simulink model "Tractor_KRAKER_etrailer_v1_2023a"  (R2023a)
settings: Solver=VariableStepAuto  StartTime=0.0  StopTime=tmax  FixedStep=dt  RelTol=1e-3  EnableMultiTasking=on
PreLoadFcn:
  | init_vehicle
  | SIMSCAPE_BE_driveline_etrailer_parameters
StartFcn:
  | tic
StopFcn:
  | toc
  | sim_stop_function
  | Etrailer_Simscape_MBM_plotting
undefined symbols (not defined in the file): brake_input, chassis_length, end_val, energyCapacity, final_x, final_y, Floor, front_overhang, initialSOC, InputSwitch, kI, L_0f, LD, mass_trailer, massload, MaxTrqOut, pose_t0, sp_t, steer_input, steer_path, steer_ratio, steer_sens, throttle_input, tire_param_drive, tire_param_steer, tire_param_trailer, tire_width, v_0, Voc, Vx, Vx_input, wheelbase, X, Y, Z
libraries: sm_lib x367, nesl_utility x280, fl_lib x15, sdl_lib x2, robotalgslib x1, simulink_extras x1, batteryecm_lib x1, ee_lib x1, BatteryEstimators x1, simulink x1, slpidlib x1, CommercialVehicleLibrary2G x1
(part 5 of 12)

== system Tractor_KRAKER_etrailer_v1_2023a/Tractor_semitrailer /Kraker etrailer/Trailer_torsion ==
  Align_Torsion joint : sm_lib/Frames and Transforms/Rigid Transform  TranslationMethod=None  TranslationStandardOffset=0  TranslationStandardOffsetUnits=m  TranslationStandardAxis=+Z  TranslationCartesianOffset=[-0.5*l 0 0]  TranslationCartesianOffsetUnits=m  TranslationROffset=0  TranslationROffsetUnits=m  TranslationZOffset=0  TranslationZOffsetUnits=m  TranslationThetaOffset=0  TranslationThetaOffsetUnits=deg  RotationMethod=AlignedAxes  RotationAngleUnits=deg  RotationStandardAxis=+Z  RotationAngle=0.0  RotationArbitraryAxis=[0 0 1]  FollAlignAxisA=+X  BaseAlignAxisA=+Z  FollAlignAxisB=+Y  BaseAlignAxisB=+Y  RotationSequenceAxes=FollowerAxes  RotationSequence=XYX  RotationSequenceAngles=[0 0 0]  RotationSequenceAnglesUnits=deg  RotationMatrix=[1 0 0; 0 1 0; 0 0 1]  Quaternion=[1 0 0 0]
  Bus Creator1 : BusCreator  Inputs=3
  Chassis rear pos : sm_lib/Frames and Transforms/Rigid Transform  TranslationMethod=Cartesian  TranslationStandardOffset=2.02-0.08  TranslationStandardOffsetUnits=m  TranslationStandardAxis=-X  TranslationCartesianOffset=[-xrev1+xcg2 0 0]  TranslationCartesianOffsetUnits=m  TranslationROffset=0  TranslationROffsetUnits=m  TranslationZOffset=0  TranslationZOffsetUnits=m  TranslationThetaOffset=0  TranslationThetaOffsetUnits=deg  RotationMethod=None  RotationAngleUnits=deg  RotationStandardAxis=+Z  RotationAngle=0.0  RotationArbitraryAxis=[0 0 1]  FollAlignAxisA=+X  BaseAlignAxisA=+Y  FollAlignAxisB=+Y  BaseAlignAxisB=+Z  RotationSequenceAxes=FollowerAxes  RotationSequence=XYX  RotationSequenceAngles=[0 0 0]  RotationSequenceAnglesUnits=deg  RotationMatrix=[1 0 0; 0 1 0; 0 0 1]  Quaternion=[1 0 0 0]
  PS-Simulink Converter - in rad : nesl_utility/PS-Simulink Converter  PhysicalDomain=network_engine_domain  SubClassName=ps_output  LeftPortType=input  RightPortType=output  PseudoPeriodic=off  Frequencies=[]  VectorFormat=1-D array  Unit=rad  AffineConversion=off
  PS-Simulink Converter4 : nesl_utility/PS-Simulink Converter  PhysicalDomain=network_engine_domain  SubClassName=ps_output  LeftPortType=input  RightPortType=output  PseudoPeriodic=off  Frequencies=[]  VectorFormat=1-D array  Unit=1  AffineConversion=off
  Realign_Torsion joint : sm_lib/Frames and Transforms/Rigid Transform  TranslationMethod=None  TranslationStandardOffset=0  TranslationStandardOffsetUnits=m  TranslationStandardAxis=+Z  TranslationCartesianOffset=[0 0 0.5*l]  TranslationCartesianOffsetUnits=m  TranslationROffset=0  TranslationROffsetUnits=m  TranslationZOffset=0  TranslationZOffsetUnits=m  TranslationThetaOffset=0  TranslationThetaOffsetUnits=deg  RotationMethod=AlignedAxes  RotationAngleUnits=deg  RotationStandardAxis=+Z  RotationAngle=0.0  RotationArbitraryAxis=[0 0 1]  FollAlignAxisA=+Z  BaseAlignAxisA=+X  FollAlignAxisB=+Y  BaseAlignAxisB=+Y  RotationSequenceAxes=FollowerAxes  RotationSequence=XYX  RotationSequenceAngles=[0 0 0]  RotationSequenceAnglesUnits=deg  RotationMatrix=[1 0 0; 0 1 0; 0 0 1]  Quaternion=[1 0 0 0]
  Subsystem : Subsystem
  Torsion Joint : sm_lib/Joints/Revolute Joint  JointMode=Normal  SenseConstraintForce=off  SenseConstraintForceX=off  SenseConstraintForceY=off  SenseConstraintForceZ=off  SenseConstraintTorque=off  SenseConstraintTorqueX=off  SenseConstraintTorqueY=off  SenseConstraintTorqueZ=off  SenseTotalForce=off  SenseTotalForceX=off  SenseTotalForceY=off  SenseTotalForceZ=off  SenseTotalTorque=off  SenseTotalTorqueX=off  SenseTotalTorqueY=off  SenseTotalTorqueZ=off  CompositeWrenchDir=FollowerOnBase  CompositeWrenchFrame=BaseFrame  EquilibriumPosition=0  EquilibriumPositionUnits=deg  SpringStiffness=800000  SpringStiffnessUnits=N*m/rad  DampingCoefficient=0  DampingCoefficientUnits=N*m/(deg/s)  TorqueActuationMode=NoTorque  MotionActuationMode=ComputedMotion  SensePosition=on  SenseVelocity=off  SenseAcceleration=off  SenseTorqueForce=off  SenseLowerLimitTorqueForce=off  SenseUpperLimitTorqueForce=off  LowerLimitSpecify=off  LowerLimitBound=-90  LowerLimitBoundUnits=deg  LowerLimitStiffness=1e4  LowerLimitStiffnessUnits=N*m/deg  LowerLimitDamping=10  LowerLimitDampingUnits=N*m/(deg/s)  LowerLimitTransitionRegionWidth=0.1  LowerLimitTransitionRegionWidthUnits=deg  UpperLimitSpecify=off  UpperLimitBound=90  UpperLimitBoundUnits=deg  UpperLimitStiffness=1e4  UpperLimitStiffnessUnits=N*m/deg  UpperLimitDamping=10  UpperLimitDampingUnits=N*m/(deg/s)  UpperLimitTransitionRegionWidth=0.1  UpperLimitTransitionRegionWidthUnits=deg  PositionTargetSpecify=off  PositionTargetPriority=High  PositionTargetValue=0  PositionTargetValueUnits=deg  VelocityTargetSpecify=off  VelocityTargetPriority=High  VelocityTargetValue=0  VelocityTargetValueUnits=deg/s
  Torsion pos : sm_lib/Frames and Transforms/Rigid Transform  TranslationMethod=Cartesian  TranslationStandardOffset=0  TranslationStandardOffsetUnits=m  TranslationStandardAxis=+Z  TranslationCartesianOffset=[(-xcg1+xrev1) 0 0]  TranslationCartesianOffsetUnits=m  TranslationROffset=0  TranslationROffsetUnits=m  TranslationZOffset=0  TranslationZOffsetUnits=m  TranslationThetaOffset=0  TranslationThetaOffsetUnits=deg  RotationMethod=None  RotationAngleUnits=deg  RotationStandardAxis=+Z  RotationAngle=0.0  RotationArbitraryAxis=[0 0 1]  FollAlignAxisA=+X  BaseAlignAxisA=+Y  FollAlignAxisB=+Y  BaseAlignAxisB=+Z  RotationSequenceAxes=FollowerAxes  RotationSequence=XYX  RotationSequenceAngles=[0 0 0]  RotationSequenceAnglesUnits=deg  RotationMatrix=[1 0 0; 0 1 0; 0 0 1]  Quaternion=[1 0 0 0]
  Transform Sensor1 : sm_lib/Frames and Transforms/Transform Sensor  MeasurementFrame=World  RotationSequence=XYX  SenseAngle=off  SenseAxis=off  SenseQ=off  SenseR=on  SenseRotationSequence=off  SenseOmegaX=off  SenseOmegaY=off  SenseOmegaZ=off  SenseQDot=off  SenseRDot=off  SenseRotationSequenceDot=off  SenseAlphaX=off  SenseAlphaY=off  SenseAlphaZ=off  SenseQDDot=off  SenseRDDot=off  SenseX=off  SenseY=off  SenseZ=off  SenseRad=off  SenseAzim=off  SenseDist=off  SenseInc=off  SenseXDot=off  SenseYDot=off  SenseZDot=off  SenseRadDot=off  SenseAzimDot=off  SenseDistDot=off  SenseIncDot=off  SenseXDDot=off  SenseYDDot=off  SenseZDDot=off  SenseRadDDot=off  SenseAzimDDot=off  SenseDistDDot=off  SenseIncDDot=off
  World Frame : sm_lib/Frames and Transforms/World Frame
  Chassis_front : PMIOPort  Side=Left
  Chassis_rear : PMIOPort  Port=2  Side=Right
  Signals : Outport
  signals : Outport  Port=2
  wires:
  PS-Simulink Converter - in rad/1 -> Signals/1
  PS-Simulink Converter4/1 -> Subsystem/1(In1)
  Bus Creator1/1 -> signals/1
  Subsystem/3(roll) -> Bus Creator1/3
  Subsystem/2(pitch) -> Bus Creator1/2
  Subsystem/1(yaw) -> Bus Creator1/1
  connections:
  Torsion pos/LConn1 -- Chassis_front/RConn1
  Chassis rear pos/RConn1 -- Chassis_rear/RConn1
  Realign_Torsion joint/RConn1 -- Chassis rear pos/LConn1
  Align_Torsion joint/RConn1 -- Torsion Joint/LConn1
  Realign_Torsion joint/LConn1 -- Torsion Joint/RConn1
  Align_Torsion joint/LConn1 -- Transform Sensor1/RConn1 -- Torsion pos/RConn1
  Torsion Joint/RConn2 -- PS-Simulink Converter - in rad/LConn1
  PS-Simulink Converter4/LConn1 -- Transform Sensor1/RConn2
  World Frame/RConn1 -- Transform Sensor1/LConn1

== system Tractor_KRAKER_etrailer_v1_2023a/Tractor_semitrailer /To_workspace_semitrailer/Fx Subsystem ==
  In1 : Inport
  Bus Selector24 : BusSelector  OutputSignals=axle1.Tire_L.Longitudinal: Fx,axle1.Tire_R.Longitudinal: Fx,axle2.Tire_L.Longitudinal: Fx,axle2.Tire_R.Longitudinal: Fx,axle3.Tire_L.Longitudinal: Fx,axle3.Tire_R.Longitudinal: Fx
  Mux : Mux  Inputs=6
  Out1 : Outport
  wires:
  In1/1 -> Bus Selector24/1
  Mux/1 -> Out1/1
  Bus Selector24/1 -> Mux/1  "<Longitudinal: Fx>"
  Bus Selector24/2 -> Mux/2  "<Longitudinal: Fx>"
  Bus Selector24/3 -> Mux/3  "<Longitudinal: Fx>"
  Bus Selector24/4 -> Mux/4  "<Longitudinal: Fx>"
  Bus Selector24/5 -> Mux/5  "<Longitudinal: Fx>"
  Bus Selector24/6 -> Mux/6  "<Longitudinal: Fx>"

== system Tractor_KRAKER_etrailer_v1_2023a/Tractor_semitrailer /To_workspace_semitrailer/Fy Subsystem ==
  In1 : Inport
  Bus Selector24 : BusSelector  OutputSignals=axle1.Tire_L.Lateral: Fy,axle1.Tire_R.Lateral: Fy,axle2.Tire_L.Lateral: Fy,axle2.Tire_R.Lateral: Fy,axle3.Tire_L.Lateral: Fy,axle3.Tire_R.Lateral: Fy
  Mux : Mux  Inputs=6
  Out1 : Outport
  wires:
  Bus Selector24/6 -> Mux/6  "<Lateral: Fy>"
  Bus Selector24/5 -> Mux/5  "<Lateral: Fy>"
  Bus Selector24/4 -> Mux/4  "<Lateral: Fy>"
  Bus Selector24/3 -> Mux/3  "<Lateral: Fy>"
  Bus Selector24/2 -> Mux/2  "<Lateral: Fy>"
  Bus Selector24/1 -> Mux/1  "<Lateral: Fy>"
  In1/1 -> Bus Selector24/1
  Mux/1 -> Out1/1

== system Tractor_KRAKER_etrailer_v1_2023a/Tractor_semitrailer /To_workspace_semitrailer/Fz Subsystem ==
  In1 : Inport
  Bus Selector24 : BusSelector  OutputSignals=axle1.Tire_L.Normal: Fz,axle1.Tire_R.Normal: Fz,axle2.Tire_L.Normal: Fz,axle2.Tire_R.Normal: Fz,axle3.Tire_L.Normal: Fz,axle3.Tire_R.Normal: Fz
  Mux : Mux  Inputs=6
  Out1 : Outport
  wires:
  Mux/1 -> Out1/1
  In1/1 -> Bus Selector24/1
  Bus Selector24/1 -> Mux/1  "<Normal: Fz>"
  Bus Selector24/2 -> Mux/2  "<Normal: Fz>"
  Bus Selector24/3 -> Mux/3  "<Normal: Fz>"
  Bus Selector24/4 -> Mux/4  "<Normal: Fz>"
  Bus Selector24/5 -> Mux/5  "<Normal: Fz>"
  Bus Selector24/6 -> Mux/6  "<Normal: Fz>"

== system Tractor_KRAKER_etrailer_v1_2023a/Tractor_semitrailer /To_workspace_semitrailer/Mz Subsystem ==
  In1 : Inport
  Bus Selector24 : BusSelector  OutputSignals=axle1.Tire_L.Aligning: Mz,axle1.Tire_R.Aligning: Mz,axle2.Tire_L.Aligning: Mz,axle2.Tire_R.Aligning: Mz,axle3.Tire_L.Aligning: Mz,axle3.Tire_R.Aligning: Mz
  Mux : Mux  Inputs=6
  Out1 : Outport
  wires:
  Mux/1 -> Out1/1
  In1/1 -> Bus Selector24/1
  Bus Selector24/1 -> Mux/1  "<Aligning: Mz>"
  Bus Selector24/2 -> Mux/2  "<Aligning: Mz>"
  Bus Selector24/3 -> Mux/3  "<Aligning: Mz>"
  Bus Selector24/4 -> Mux/4  "<Aligning: Mz>"
  Bus Selector24/5 -> Mux/5  "<Aligning: Mz>"
  Bus Selector24/6 -> Mux/6  "<Aligning: Mz>"

== system Tractor_KRAKER_etrailer_v1_2023a/Tractor_semitrailer /To_workspace_semitrailer/Omega Subsystem ==
  In1 : Inport
  Bus Selector6 : BusSelector  OutputSignals=axle1.Omega1,axle1.Omega2,axle2.Omega1,axle2.Omega2,axle3.Omega1,axle3.Omega2
  Mux : Mux  Inputs=6
  Out1 : Outport
  wires:
  Bus Selector6/6 -> Mux/6  "<Omega2>"
  Bus Selector6/5 -> Mux/5  "<Omega1>"
  Bus Selector6/4 -> Mux/4  "<Omega2>"
  Bus Selector6/3 -> Mux/3  "<Omega1>"
  Bus Selector6/2 -> Mux/2  "<Omega2>"
  Bus Selector6/1 -> Mux/1  "<Omega1>"
  Mux/1 -> Out1/1
  In1/1 -> Bus Selector6/1

== system Tractor_KRAKER_etrailer_v1_2023a/Tractor_semitrailer /To_workspace_tractor/Fx Subsystem ==
  In : Inport
  Bus Selector24 : BusSelector  OutputSignals=steeraxle.Tire1_L.Longitudinal: Fx,steeraxle.Tire1_R.Longitudinal: Fx,driveaxle.Tire1_L.Longitudinal: Fx,driveaxle.Tire1_R.Longitudinal: Fx,driveaxle.Tire2_L.Longitudinal: Fx,driveaxle.Tire2_R.Longitudinal: Fx
  Mux : Mux  Inputs=6
  Out : Outport
  wires:
  In/1 -> Bus Selector24/1
  Mux/1 -> Out/1
  Bus Selector24/1 -> Mux/1  "<Longitudinal: Fx>"
  Bus Selector24/2 -> Mux/2  "<Longitudinal: Fx>"
  Bus Selector24/3 -> Mux/3  "<Longitudinal: Fx>"
  Bus Selector24/4 -> Mux/4  "<Longitudinal: Fx>"
  Bus Selector24/5 -> Mux/5  "<Longitudinal: Fx>"
  Bus Selector24/6 -> Mux/6  "<Longitudinal: Fx>"

== system Tractor_KRAKER_etrailer_v1_2023a/Tractor_semitrailer /To_workspace_tractor/Fy Subsystem ==
  In1 : Inport
  Bus Selector24 : BusSelector  OutputSignals=steeraxle.Tire1_L.Lateral: Fy,steeraxle.Tire1_R.Lateral: Fy,driveaxle.Tire1_L.Lateral: Fy,driveaxle.Tire1_R.Lateral: Fy,driveaxle.Tire2_L.Lateral: Fy,driveaxle.Tire2_R.Lateral: Fy
  Mux : Mux  Inputs=6
  Out1 : Outport
  wires:
  In1/1 -> Bus Selector24/1
  Mux/1 -> Out1/1
  Bus Selector24/1 -> Mux/1  "<Lateral: Fy>"
  Bus Selector24/2 -> Mux/2  "<Lateral: Fy>"
  Bus Selector24/3 -> Mux/3  "<Lateral: Fy>"
  Bus Selector24/4 -> Mux/4  "<Lateral: Fy>"
  Bus Selector24/5 -> Mux/5  "<Lateral: Fy>"
  Bus Selector24/6 -> Mux/6  "<Lateral: Fy>"

== system Tractor_KRAKER_etrailer_v1_2023a/Tractor_semitrailer /To_workspace_tractor/Fz Subsystem ==
  In1 : Inport
  Bus Selector24 : BusSelector  OutputSignals=steeraxle.Tire1_L.Normal: Fz,steeraxle.Tire1_R.Normal: Fz,driveaxle.Tire1_L.Normal: Fz,driveaxle.Tire1_R.Normal: Fz,driveaxle.Tire2_L.Normal: Fz,driveaxle.Tire2_R.Normal: Fz
  Mux : Mux  Inputs=6
  Out1 : Outport
  wires:
  In1/1 -> Bus Selector24/1
  Mux/1 -> Out1/1
  Bus Selector24/1 -> Mux/1  "<Normal: Fz>"
  Bus Selector24/2 -> Mux/2  "<Normal: Fz>"
  Bus Selector24/3 -> Mux/3  "<Normal: Fz>"
  Bus Selector24/4 -> Mux/4  "<Normal: Fz>"
  Bus Selector24/5 -> Mux/5  "<Normal: Fz>"
  Bus Selector24/6 -> Mux/6  "<Normal: Fz>"

== system Tractor_KRAKER_etrailer_v1_2023a/Tractor_semitrailer /To_workspace_tractor/Mz Subsystem ==
  In1 : Inport
  Bus Selector24 : BusSelector  OutputSignals=steeraxle.Tire1_L.Aligning: Mz,steeraxle.Tire1_R.Aligning: Mz,driveaxle.Tire1_L.Aligning: Mz,driveaxle.Tire1_R.Aligning: Mz,driveaxle.Tire2_L.Aligning: Mz,driveaxle.Tire2_R.Aligning: Mz
  Mux : Mux  Inputs=6
  Out1 : Outport
  wires:
  In1/1 -> Bus Selector24/1
  Bus Selector24/6 -> Mux/6  "<Aligning: Mz>"
  Mux/1 -> Out1/1
  Bus Selector24/5 -> Mux/5  "<Aligning: Mz>"
  Bus Selector24/1 -> Mux/1  "<Aligning: Mz>"
  Bus Selector24/3 -> Mux/3  "<Aligning: Mz>"
  Bus Selector24/4 -> Mux/4  "<Aligning: Mz>"
  Bus Selector24/2 -> Mux/2  "<Aligning: Mz>"

== system Tractor_KRAKER_etrailer_v1_2023a/Tractor_semitrailer /To_workspace_tractor/Omega Subsystem ==
  In1 : Inport
  Bus Selector6 : BusSelector  OutputSignals=steeraxle.Omega1,steeraxle.Omega2,driveaxle.Omega1,driveaxle.Omega2
  Mux : Mux
  Out1 : Outport
  wires:
  Bus Selector6/2 -> Mux/2  "<Omega2>"
  Bus Selector6/4 -> Mux/4  "<Omega2>"
  Bus Selector6/3 -> Mux/3  "<Omega1>"
  Bus Selector6/1 -> Mux/1  "<Omega1>"
  Mux/1 -> Out1/1
  In1/1 -> Bus Selector6/1

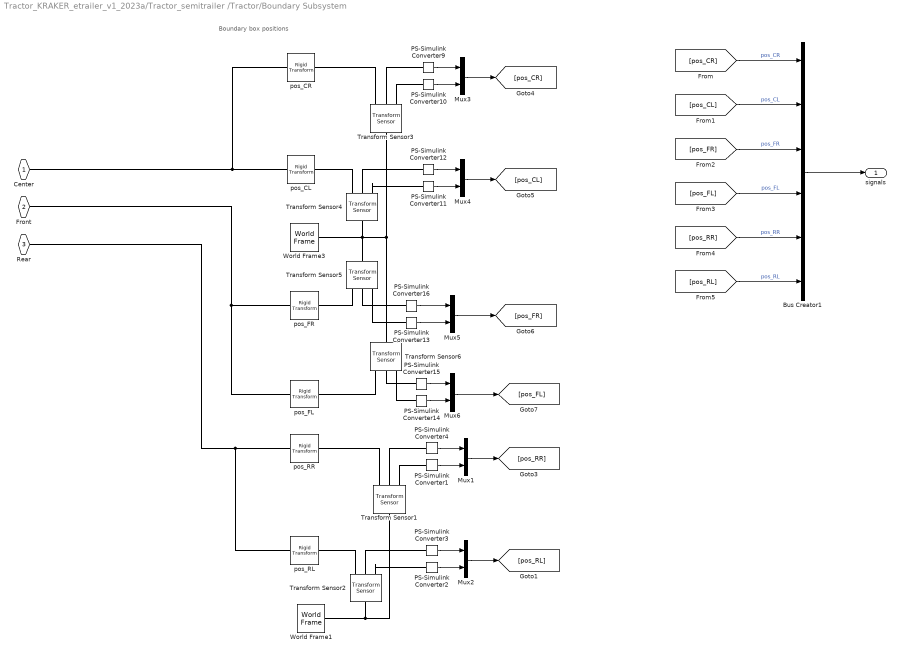
== system Tractor_KRAKER_etrailer_v1_2023a/Tractor_semitrailer /Tractor/Boundary Subsystem ==
  note: Boundary box positions
  Bus Creator1 : BusCreator  Inputs=6
  Mux{1..6} (6 alike) : Mux  Inputs=2
  PS-Simulink Converter{1..4,9..16} (12 alike) : nesl_utility/PS-Simulink Converter  PhysicalDomain=network_engine_domain  SubClassName=ps_output  LeftPortType=input  RightPortType=output  PseudoPeriodic=off  Frequencies=[]  VectorFormat=1-D array  Unit=inherit  AffineConversion=off
  Transform Sensor{1..6} (6 alike) : sm_lib/Frames and Transforms/Transform Sensor  MeasurementFrame=World  RotationSequence=XYX  SenseAngle=off  SenseAxis=off  SenseQ=off  SenseR=off  SenseRotationSequence=off  SenseOmegaX=off  SenseOmegaY=off  SenseOmegaZ=off  SenseQDot=off  SenseRDot=off  SenseRotationSequenceDot=off  SenseAlphaX=off  SenseAlphaY=off  SenseAlphaZ=off  SenseQDDot=off  SenseRDDot=off  SenseX=on  SenseY=on  SenseZ=off  SenseRad=off  SenseAzim=off  SenseDist=off  SenseInc=off  SenseXDot=off  SenseYDot=off  SenseZDot=off  SenseRadDot=off  SenseAzimDot=off  SenseDistDot=off  SenseIncDot=off  SenseXDDot=off  SenseYDDot=off  SenseZDDot=off  SenseRadDDot=off  SenseAzimDDot=off  SenseDistDDot=off  SenseIncDDot=off
  World Frame1 : sm_lib/Frames and Transforms/World Frame
  World Frame3 : sm_lib/Frames and Transforms/World Frame
  pos_CL : sm_lib/Frames and Transforms/Rigid Transform  TranslationMethod=Cartesian  TranslationStandardOffset=0  TranslationStandardOffsetUnits=m  TranslationStandardAxis=+Z  TranslationCartesianOffset=[0 1.25 -h1/2]  TranslationCartesianOffsetUnits=m  TranslationROffset=0  TranslationROffsetUnits=m  TranslationZOffset=0  TranslationZOffsetUnits=m  TranslationThetaOffset=0  TranslationThetaOffsetUnits=deg  RotationMethod=None  RotationAngleUnits=deg  RotationStandardAxis=+Z  RotationAngle=0.0  RotationArbitraryAxis=[0 0 1]  FollAlignAxisA=+X  BaseAlignAxisA=+Y  FollAlignAxisB=+Y  BaseAlignAxisB=+Z  RotationSequenceAxes=FollowerAxes  RotationSequence=XYX  RotationSequenceAngles=[0 0 0]  RotationSequenceAnglesUnits=deg  RotationMatrix=[1 0 0; 0 1 0; 0 0 1]  Quaternion=[1 0 0 0]
  pos_CR : sm_lib/Frames and Transforms/Rigid Transform  TranslationMethod=Cartesian  TranslationStandardOffset=0  TranslationStandardOffsetUnits=m  TranslationStandardAxis=+Z  TranslationCartesianOffset=[0 -1.25 -h1/2]  TranslationCartesianOffsetUnits=m  TranslationROffset=0  TranslationROffsetUnits=m  TranslationZOffset=0  TranslationZOffsetUnits=m  TranslationThetaOffset=0  TranslationThetaOffsetUnits=deg  RotationMethod=None  RotationAngleUnits=deg  RotationStandardAxis=+Z  RotationAngle=0.0  RotationArbitraryAxis=[0 0 1]  FollAlignAxisA=+X  BaseAlignAxisA=+Y  FollAlignAxisB=+Y  BaseAlignAxisB=+Z  RotationSequenceAxes=FollowerAxes  RotationSequence=XYX  RotationSequenceAngles=[0 0 0]  RotationSequenceAnglesUnits=deg  RotationMatrix=[1 0 0; 0 1 0; 0 0 1]  Quaternion=[1 0 0 0]
  pos_FL : sm_lib/Frames and Transforms/Rigid Transform  TranslationMethod=Cartesian  TranslationStandardOffset=0  TranslationStandardOffsetUnits=m  TranslationStandardAxis=+Z  TranslationCartesianOffset=[0 1.25 -h1/2]  TranslationCartesianOffsetUnits=m  TranslationROffset=0  TranslationROffsetUnits=m  TranslationZOffset=0  TranslationZOffsetUnits=m  TranslationThetaOffset=0  TranslationThetaOffsetUnits=deg  RotationMethod=None  RotationAngleUnits=deg  RotationStandardAxis=+Z  RotationAngle=0.0  RotationArbitraryAxis=[0 0 1]  FollAlignAxisA=+X  BaseAlignAxisA=+Y  FollAlignAxisB=+Y  BaseAlignAxisB=+Z  RotationSequenceAxes=FollowerAxes  RotationSequence=XYX  RotationSequenceAngles=[0 0 0]  RotationSequenceAnglesUnits=deg  RotationMatrix=[1 0 0; 0 1 0; 0 0 1]  Quaternion=[1 0 0 0]
  pos_FR : sm_lib/Frames and Transforms/Rigid Transform  TranslationMethod=Cartesian  TranslationStandardOffset=0  TranslationStandardOffsetUnits=m  TranslationStandardAxis=+Z  TranslationCartesianOffset=[0 -1.25 -h1/2]  TranslationCartesianOffsetUnits=m  TranslationROffset=0  TranslationROffsetUnits=m  TranslationZOffset=0  TranslationZOffsetUnits=m  TranslationThetaOffset=0  TranslationThetaOffsetUnits=deg  RotationMethod=None  RotationAngleUnits=deg  RotationStandardAxis=+Z  RotationAngle=0.0  RotationArbitraryAxis=[0 0 1]  FollAlignAxisA=+X  BaseAlignAxisA=+Y  FollAlignAxisB=+Y  BaseAlignAxisB=+Z  RotationSequenceAxes=FollowerAxes  RotationSequence=XYX  RotationSequenceAngles=[0 0 0]  RotationSequenceAnglesUnits=deg  RotationMatrix=[1 0 0; 0 1 0; 0 0 1]  Quaternion=[1 0 0 0]
  pos_RL : sm_lib/Frames and Transforms/Rigid Transform  TranslationMethod=Cartesian  TranslationStandardOffset=0  TranslationStandardOffsetUnits=m  TranslationStandardAxis=+Z  TranslationCartesianOffset=[0 1.25 -h2/2]  TranslationCartesianOffsetUnits=m  TranslationROffset=0  TranslationROffsetUnits=m  TranslationZOffset=0  TranslationZOffsetUnits=m  TranslationThetaOffset=0  TranslationThetaOffsetUnits=deg  RotationMethod=None  RotationAngleUnits=deg  RotationStandardAxis=+Z  RotationAngle=0.0  RotationArbitraryAxis=[0 0 1]  FollAlignAxisA=+X  BaseAlignAxisA=+Y  FollAlignAxisB=+Y  BaseAlignAxisB=+Z  RotationSequenceAxes=FollowerAxes  RotationSequence=XYX  RotationSequenceAngles=[0 0 0]  RotationSequenceAnglesUnits=deg  RotationMatrix=[1 0 0; 0 1 0; 0 0 1]  Quaternion=[1 0 0 0]
  pos_RR : sm_lib/Frames and Transforms/Rigid Transform  TranslationMethod=Cartesian  TranslationStandardOffset=0  TranslationStandardOffsetUnits=m  TranslationStandardAxis=+Z  TranslationCartesianOffset=[0 -1.25 -h2/2]  TranslationCartesianOffsetUnits=m  TranslationROffset=0  TranslationROffsetUnits=m  TranslationZOffset=0  TranslationZOffsetUnits=m  TranslationThetaOffset=0  TranslationThetaOffsetUnits=deg  RotationMethod=None  RotationAngleUnits=deg  RotationStandardAxis=+Z  RotationAngle=0.0  RotationArbitraryAxis=[0 0 1]  FollAlignAxisA=+X  BaseAlignAxisA=+Y  FollAlignAxisB=+Y  BaseAlignAxisB=+Z  RotationSequenceAxes=FollowerAxes  RotationSequence=XYX  RotationSequenceAngles=[0 0 0]  RotationSequenceAnglesUnits=deg  RotationMatrix=[1 0 0; 0 1 0; 0 0 1]  Quaternion=[1 0 0 0]
  Center : PMIOPort  Side=Right
  Front : PMIOPort  Port=2  Side=Right
  Rear : PMIOPort  Port=3  Side=Right
  signals : Outport
  wires:
  PS-Simulink Converter13/1 -> Mux5/2
  PS-Simulink Converter10/1 -> Mux3/2
  PS-Simulink Converter16/1 -> Mux5/1
  Mux6/1 -> [pos_FL]
  PS-Simulink Converter15/1 -> Mux6/1
  PS-Simulink Converter14/1 -> Mux6/2
  Mux5/1 -> [pos_FR]
  PS-Simulink Converter9/1 -> Mux3/1
  Mux3/1 -> [pos_CR]
  PS-Simulink Converter11/1 -> Mux4/2
  PS-Simulink Converter12/1 -> Mux4/1
  Mux4/1 -> [pos_CL]
  PS-Simulink Converter1/1 -> Mux1/2
  Mux2/1 -> [pos_RL]
  Mux1/1 -> [pos_RR]
  PS-Simulink Converter3/1 -> Mux2/1
  PS-Simulink Converter2/1 -> Mux2/2
  PS-Simulink Converter4/1 -> Mux1/1
  [pos_RL] -> Bus Creator1/6  "pos_RL"
  [pos_RR] -> Bus Creator1/5  "pos_RR"
  [pos_FL] -> Bus Creator1/4  "pos_FL"
  [pos_FR] -> Bus Creator1/3  "pos_FR"
  [pos_CL] -> Bus Creator1/2  "pos_CL"
  [pos_CR] -> Bus Creator1/1  "pos_CR"
  Bus Creator1/1 -> signals/1
  connections:
  Transform Sensor6/LConn1 -- Transform Sensor3/LConn1 -- Transform Sensor5/LConn1 -- Transform Sensor4/LConn1 -- World Frame3/RConn1
  pos_FR/LConn1 -- Front/RConn1 -- pos_FL/LConn1
  pos_CL/LConn1 -- Center/RConn1 -- pos_CR/LConn1
  Transform Sensor3/RConn1 -- pos_CR/RConn1
  Transform Sensor5/RConn1 -- pos_FR/RConn1
  Transform Sensor6/RConn1 -- pos_FL/RConn1
  Transform Sensor4/RConn3 -- PS-Simulink Converter11/LConn1
  Transform Sensor4/RConn2 -- PS-Simulink Converter12/LConn1
  Transform Sensor5/RConn2 -- PS-Simulink Converter16/LConn1
  Transform Sensor6/RConn3 -- PS-Simulink Converter14/LConn1
  Transform Sensor6/RConn2 -- PS-Simulink Converter15/LConn1
  Transform Sensor3/RConn3 -- PS-Simulink Converter10/LConn1
  Transform Sensor3/RConn2 -- PS-Simulink Converter9/LConn1
  Transform Sensor5/RConn3 -- PS-Simulink Converter13/LConn1
  Transform Sensor4/RConn1 -- pos_CL/RConn1
  pos_RL/LConn1 -- Rear/RConn1 -- pos_RR/LConn1
  Transform Sensor1/LConn1 -- Transform Sensor2/LConn1 -- World Frame1/RConn1
  Transform Sensor2/RConn1 -- pos_RL/RConn1
  Transform Sensor1/RConn1 -- pos_RR/RConn1
  Transform Sensor2/RConn2 -- PS-Simulink Converter3/LConn1
  Transform Sensor1/RConn2 -- PS-Simulink Converter4/LConn1
  Transform Sensor1/RConn3 -- PS-Simulink Converter1/LConn1
  Transform Sensor2/RConn3 -- PS-Simulink Converter2/LConn1

== system Tractor_KRAKER_etrailer_v1_2023a/Tractor_semitrailer /Tractor/Braking system ==
  input (0-1) : Inport
  DriveTrqs_etrailer : Inport  Port=2
  Abs : Abs  SaturateOnIntegerOverflow=off
  Add : Sum
  Add1 : Sum  Inputs=+++
  Add2 : Sum  Inputs=+++
  Bus Selector : BusSelector  OutputSignals=DriveTrqR,DriveTrqL
  MATLAB Function : MATLAB Function  TreatAsAtomicUnit=on
  Mux{,1..7} (8 alike) : Mux  Inputs=2
  Saturation : Saturate  UpperLimit=1  LowerLimit=0
  Saturation1 : Saturate  UpperLimit=0  LowerLimit=-inf
  Scope : Scope  NumInputPorts=2
  Scope1 : Scope
  Terminator : Terminator
  Terminator1 : Terminator
  Terminator2 : Terminator
  brake moment gain1 : Gain  Gain=20000  SaturateOnIntegerOverflow=on  OutDataTypeStr=Inherit: Same as input  ParamDataTypeStr=Inherit: Same as input
  brake moment gain2 : Gain  Gain=28000  SaturateOnIntegerOverflow=on  OutDataTypeStr=Inherit: Same as input  ParamDataTypeStr=Inherit: Same as input
  brake moment gain3 : Gain  Gain=15000  SaturateOnIntegerOverflow=on  OutDataTypeStr=Inherit: Same as input  ParamDataTypeStr=Inherit: Same as input
  Mb_rear : Outport  VectorParamsAs1DForOutWhenUnconnected=off
  Mb_front : Outport  Port=2  VectorParamsAs1DForOutWhenUnconnected=off
  Mb_trailer : Outport  Port=3  VectorParamsAs1DForOutWhenUnconnected=off
  wires:
  brake moment gain1/1 -> Add1/1, Mux2/1, Mux2/2
  brake moment gain2/1 -> Add1/2, Mux1/1, Mux1/2
  input (0-1)/1 -> Saturation/1
  brake moment gain3/1 -> Add1/3, Mux/1, Mux/2
  Saturation/1 -> brake moment gain1/1, brake moment gain2/1, brake moment gain3/1
  DriveTrqs_etrailer/1 -> Bus Selector/1
  Bus Selector/2 -> Add/2  "<DriveTrqL>"
  Bus Selector/1 -> Add/1  "<DriveTrqR>"
  Add/1 -> Saturation1/1
  Add1/1 -> Mux7/1, Mux6/1, MATLAB Function/1(Sum_brake_tractor)  "Sum_brake_Tractor"
  Saturation1/1 -> Abs/1
  Abs/1 -> Mux6/2, MATLAB Function/2(sum_brake_etrailer)  "Sum_brake_Etrailer"
  MATLAB Function/1(Mb_front) -> Add2/1, Mux3/2, Mux3/1
  Mux3/1 -> Mb_front/1
  MATLAB Function/2(Mb_rear) -> Add2/2, Mux4/1, Mux4/2
  Mux4/1 -> Mb_rear/1
  MATLAB Function/3(Mb_trailer) -> Add2/3, Mux5/1, Mux5/2
  Mux5/1 -> Mb_trailer/1
  Mux/1 -> Terminator/1
  Mux1/1 -> Terminator1/1
  Mux2/1 -> Terminator2/1
  Mux6/1 -> Scope/1
  MATLAB Function/4(flag) -> Scope/2  "Flag"
  Add2/1 -> Mux7/2  "Sum_after_logic"
  Mux7/1 -> Scope1/1

== system Tractor_KRAKER_etrailer_v1_2023a/Tractor_semitrailer /Tractor/Cabin ==
  Brick Solid : sm_lib/Body Elements/Brick Solid  GraphicAmbientColor=[0.15 0.15 0.15 1.0]  BasedOnType=Density  BrickDimensions=[2 2 2.5]  BrickDimensionsUnits=m  CenterOfMass=[0 0 0]  CenterOfMassUnits=m  GraphicDiffuseColor=[0.2 1.0 0.0]  Density=1000  DensityUnits=kg/m^3  DoExposeReferenceFrame=on  GraphicEmissiveColor=[0.0 0.0 0.0 1.0]  ExportEntireGeometry=off  SerializedFrames=<Frames><Frame><Id>Frame1</Id><Value><Name>F1</Name><Origin><Source>ReferenceFrame</Source><FeatureName></FeatureName></Origin><PrimaryAxis><DefinedDirection>+Z</DefinedDirection><Source>ReferenceFrame</Source><SourceDirection>+Z</SourceDirection><FeatureName></FeatureName></PrimaryAxis><SecondaryAxis><DefinedDirection>+X</DefinedDirection><Source>ReferenceFrame</Source><SourceDirection>+X</SourceDirection><FeatureName></FeatureName></SecondaryAxis></Value></Frame></Frames>  MarkerShape=Sphere  MarkerSize=10  GraphicType=FromGeometry  InertiaType=Custom  Mass=1300  MassUnits=kg  MomentsOfInertia=[1100 1100 1100]  MomentsOfInertiaUnits=kg*m^2  GraphicOpacity=0.6  ProductsOfInertia=[0 0 0]  ProductsOfInertiaUnits=kg*m^2  GraphicShininess=75  GraphicSpecularColor=[0.5 0.5 0.5 1.0]  GraphicVisPropType=SimpleVisualProperties
  Rigid Transform2 : sm_lib/Frames and Transforms/Rigid Transform  TranslationMethod=Cartesian  TranslationStandardOffset=0  TranslationStandardOffsetUnits=m  TranslationStandardAxis=+Z  TranslationCartesianOffset=[xref-0.75 0 zref-0.9+1]  TranslationCartesianOffsetUnits=m  TranslationROffset=0  TranslationROffsetUnits=m  TranslationZOffset=0  TranslationZOffsetUnits=m  TranslationThetaOffset=0  TranslationThetaOffsetUnits=deg  RotationMethod=None  RotationAngleUnits=deg  RotationStandardAxis=+Z  RotationAngle=0.0  RotationArbitraryAxis=[0 0 1]  FollAlignAxisA=+X  BaseAlignAxisA=+Y  FollAlignAxisB=+Y  BaseAlignAxisB=+Z  RotationSequenceAxes=FollowerAxes  RotationSequence=XYX  RotationSequenceAngles=[0 0 0]  RotationSequenceAnglesUnits=deg  RotationMatrix=[1 0 0; 0 1 0; 0 0 1]  Quaternion=[1 0 0 0]
  Subsystem : Subsystem  Commented=on
      mask Display: disp('Cabin CAD Model')
  Chassis : PMIOPort  Side=Right
  connections:
  Subsystem/LConn1 -- Brick Solid/LConn1
  Chassis/RConn1 -- Rigid Transform2/LConn1
  Rigid Transform2/RConn1 -- Brick Solid/RConn1

== system Tractor_KRAKER_etrailer_v1_2023a/Tractor_semitrailer /Tractor/Cameras ==
  Front Camera Sphere : sm_lib/Body Elements/Spherical Solid  GraphicAmbientColor=[0.15 0.15 0.15 1.0]  BasedOnType=Density  CenterOfMass=[0 0 0]  CenterOfMassUnits=m  GraphicDiffuseColor=[0.5 0.5 0.5]  Density=1000  DensityUnits=kg/m^3  DoExposeReferenceFrame=on  GraphicEmissiveColor=[0.0 0.0 0.0 1.0]  ExportEntireGeometry=off  SerializedExposedGeometries=<ExposedGeometries/>  SerializedFrames=<Frames/>  MarkerShape=Sphere  MarkerSize=10  GraphicType=FromGeometry  InertiaType=PointMass  Mass=1e-09  MassUnits=kg  MomentsOfInertia=[1 1 1]  MomentsOfInertiaUnits=kg*m^2  GraphicOpacity=0  ProductsOfInertia=[0 0 0]  ProductsOfInertiaUnits=kg*m^2  GraphicShininess=75  GraphicSpecularColor=[0.5 0.5 0.5 1.0]  SphereRadius=1e-09  SphereRadiusUnits=m  GraphicVisPropType=SimpleVisualProperties
  Front Camera Transform : sm_lib/Frames and Transforms/Rigid Transform  TranslationMethod=Cartesian  TranslationStandardOffset=0  TranslationStandardOffsetUnits=m  TranslationStandardAxis=+Z  TranslationCartesianOffset=[-10 0 6]  TranslationCartesianOffsetUnits=m  TranslationROffset=0  TranslationROffsetUnits=m  TranslationZOffset=0  TranslationZOffsetUnits=m  TranslationThetaOffset=0  TranslationThetaOffsetUnits=deg  RotationMethod=None  RotationAngleUnits=deg  RotationStandardAxis=+Y  RotationAngle=90  RotationArbitraryAxis=[0 0 1]  FollAlignAxisA=+X  BaseAlignAxisA=+Y  FollAlignAxisB=+Y  BaseAlignAxisB=+Z  RotationSequenceAxes=FollowerAxes  RotationSequence=XYX  RotationSequenceAngles=[0 0 0]  RotationSequenceAnglesUnits=deg  RotationMatrix=[1 0 0; 0 1 0; 0 0 1]  Quaternion=[1 0 0 0]
  Side Camera Sphere : sm_lib/Body Elements/Spherical Solid  GraphicAmbientColor=[0.15 0.15 0.15 1.0]  BasedOnType=Density  CenterOfMass=[0 0 0]  CenterOfMassUnits=m  GraphicDiffuseColor=[0.5 0.5 0.5]  Density=1000  DensityUnits=kg/m^3  DoExposeReferenceFrame=on  GraphicEmissiveColor=[0.0 0.0 0.0 1.0]  ExportEntireGeometry=off  SerializedExposedGeometries=<ExposedGeometries/>  SerializedFrames=<Frames/>  MarkerShape=Sphere  MarkerSize=10  GraphicType=FromGeometry  InertiaType=PointMass  Mass=1e-09  MassUnits=kg  MomentsOfInertia=[1 1 1]  MomentsOfInertiaUnits=kg*m^2  GraphicOpacity=0  ProductsOfInertia=[0 0 0]  ProductsOfInertiaUnits=kg*m^2  GraphicShininess=75  GraphicSpecularColor=[0.5 0.5 0.5 1.0]  SphereRadius=1e-09  SphereRadiusUnits=m  GraphicVisPropType=SimpleVisualProperties
  Side Camera Transform : sm_lib/Frames and Transforms/Rigid Transform  TranslationMethod=Cartesian  TranslationStandardOffset=0  TranslationStandardOffsetUnits=m  TranslationStandardAxis=+Z  TranslationCartesianOffset=[5 3 3]  TranslationCartesianOffsetUnits=m  TranslationROffset=0  TranslationROffsetUnits=m  TranslationZOffset=0  TranslationZOffsetUnits=m  TranslationThetaOffset=0  TranslationThetaOffsetUnits=deg  RotationMethod=None  RotationAngleUnits=deg  RotationStandardAxis=+Z  RotationAngle=90  RotationArbitraryAxis=[0 0 1]  FollAlignAxisA=+X  BaseAlignAxisA=+Y  FollAlignAxisB=+Y  BaseAlignAxisB=+Z  RotationSequenceAxes=FollowerAxes  RotationSequence=XYX  RotationSequenceAngles=[0 0 0]  RotationSequenceAnglesUnits=deg  RotationMatrix=[1 0 0; 0 1 0; 0 0 1]  Quaternion=[1 0 0 0]
  " " : PMIOPort  Side=Left
  connections:
  Side Camera Transform/LConn1 -- Front Camera Transform/LConn1 -- " "/RConn1
  Side Camera Sphere/RConn1 -- Side Camera Transform/RConn1
  Front Camera Sphere/RConn1 -- Front Camera Transform/RConn1
